simulink model "sim_nomal_regulator"  (R2019a)
settings: Solver=FixedStepAuto  StartTime=0.0  StopTime=20  FixedStep=sT  RelTol=1e-3
InitFcn:
  | sim_param;
values from neighbouring files (symbols this model uses):
  bn = 50    [robot_param.m]    (also in sim_robot_param.m)
  bt = 50    [robot_param.m]    (also in sim_robot_param.m)
  foot_x = 0.07    [robot_param.m]    (also in sim_robot_param.m)
  foot_y = 0.045    [robot_param.m]    (also in sim_robot_param.m)
  foot_z = 0.01    [robot_param.m]    (also in sim_robot_param.m)
  height_plane = 0.025    [robot_param.m]    (also in sim_robot_param.m)
  inix = [0.00 0.00]'    [param.m]    (also in sim_param.m)
  iniXzmax = 0.05    [param.m]    (also in sim_param.m)
  iniXzmin = -0.05    [param.m]    (also in sim_param.m)
  iniy = [0.00 0.00]'    [param.m]    (also in sim_param.m)
  iniYzmax = 0.0625    [param.m]    (also in sim_param.m)
  iniYzmin = -0.0625    [param.m]    (also in sim_param.m)
  kn = 5000    [robot_param.m]    (also in sim_robot_param.m)
  kt = 5000    [robot_param.m]    (also in sim_robot_param.m)
  mu_d = 0.8    [robot_param.m]    (also in sim_robot_param.m)
  mu_s = 2    [robot_param.m]    (also in sim_robot_param.m)
  plane_x = 3    [robot_param.m]    (also in sim_robot_param.m = 6)
  plane_y = 1    [robot_param.m]    (also in sim_robot_param.m)
  R = 20    [param.m]    (also in sim_param.m = 1)
  sT = 0.02    [param.m]    (also in sim_param.m = 0.001)
  torso_offset_x = 0.0    (= 0)    [robot_param.m]    (also in sim_robot_param.m)
  torso_offset_z = -torso_z/2    (= -0.05)    [robot_param.m]    (also in sim_robot_param.m)
  torso_x = 0.1    [robot_param.m]    (also in sim_robot_param.m)
  torso_y = 0.08    [robot_param.m]    (also in sim_robot_param.m)
  torso_z = 0.10    (= 0.1)    [robot_param.m]    (also in sim_robot_param.m)
  w = sqrt(g/zc)    [param.m]    (also in sim_param.m)
  zvt = 1e-3    (= 0.001)    [robot_param.m]    (also in sim_robot_param.m)
undefined symbols (not defined in the file or in its folder): Ad, Bd, Cd, Dd, DiscIntNeverNeededParam, Discrete, sigbuilder_block, Time, X, Y, Z
libraries: nesl_utility x142, sm_lib x86, cstblocks x11, ctrlSharedLib x8
(part 5 of 6)

== system sim_nomal_regulator/simulation/Robot/Right Leg/Subsystem7 ==
  Chart : Stateflow chart  TreatAsAtomicUnit=on
  Constant1 : Constant  Value=kt
  Constant2 : Constant  Value=mu_d
  Constant3 : Constant  Value=mu_s
  Constant4 : Constant  Value=zvt
  Constant5 : Constant  Value=bt
  Constant6 : Constant  Value=bn
  Constant7 : Constant  Value=kn
  External Force and Torque : sm_lib/Forces and Torques/External Force and Torque  ForceResolutionFrame=AttachedFrame  EnableForceX=off  EnableForceY=off  EnableForceZ=off  EnableForce=on  TorqueResolutionFrame=AttachedFrame  EnableTorqueX=off  EnableTorqueY=off  EnableTorqueZ=off  EnableTorque=off
  Mux : Mux  Inputs=3
  PS-Simulink Converter1 : nesl_utility/PS-Simulink Converter  PhysicalDomain=network_engine_domain  SubClassName=ps_output  LeftPortType=input  RightPortType=output  PseudoPeriodic=off  Frequencies=[]  Unit=1  AffineConversion=off
  PS-Simulink Converter2 : nesl_utility/PS-Simulink Converter  PhysicalDomain=network_engine_domain  SubClassName=ps_output  LeftPortType=input  RightPortType=output  PseudoPeriodic=off  Frequencies=[]  Unit=1  AffineConversion=off
  PS-Simulink Converter4 : nesl_utility/PS-Simulink Converter  PhysicalDomain=network_engine_domain  SubClassName=ps_output  LeftPortType=input  RightPortType=output  PseudoPeriodic=off  Frequencies=[]  Unit=m/s  AffineConversion=off
  PS-Simulink Converter5 : nesl_utility/PS-Simulink Converter  PhysicalDomain=network_engine_domain  SubClassName=ps_output  LeftPortType=input  RightPortType=output  PseudoPeriodic=off  Frequencies=[]  Unit=m/s  AffineConversion=off
  PS-Simulink dpn : nesl_utility/PS-Simulink Converter  PhysicalDomain=network_engine_domain  SubClassName=ps_output  LeftPortType=input  RightPortType=output  PseudoPeriodic=off  Frequencies=[]  Unit=m/s  AffineConversion=off
  PS-Simulink pn : nesl_utility/PS-Simulink Converter  PhysicalDomain=network_engine_domain  SubClassName=ps_output  LeftPortType=input  RightPortType=output  PseudoPeriodic=off  Frequencies=[]  Unit=1  AffineConversion=off
  Simulink-PS Converter : nesl_utility/Simulink-PS Converter  PhysicalDomain=network_engine_domain  SubClassName=ps_input  LeftPortType=input  RightPortType=output  PseudoPeriodic=off  Frequencies=[]  NoiseDistribution=none  NoiseParameters=[]  Unit=N  AffineConversion=off  FilteringAndDerivatives=provide  SimscapeFilterOrder=1  InputFilterTimeConstant=0.001  UdotUserProvided=0
  Transform Sensor : sm_lib/Frames and Transforms/Transform Sensor  MeasurementFrame=World  SenseAngle=off  SenseAxis=off  SenseAngle1=off  SenseAngle2=off  SenseAngle3=off  SenseQ=off  SenseR=off  SenseOmegaX=off  SenseOmegaY=off  SenseOmegaZ=off  SenseOmega1=off  SenseOmega2=off  SenseOmega3=off  SenseQDot=off  SenseRDot=off  SenseAlphaX=off  SenseAlphaY=off  SenseAlphaZ=off  SenseAlpha1=off  SenseAlpha2=off  SenseAlpha3=off  SenseQDDot=off  SenseRDDot=off  SenseX=on  SenseY=on  SenseZ=on  SenseRad=off  SenseAzim=off  SenseDist=off  SenseInc=off  SenseXDot=on  SenseYDot=on  SenseZDot=on  SenseRadDot=off  SenseAzimDot=off  SenseDistDot=off  SenseIncDot=off  SenseXDDot=off  SenseYDDot=off  SenseZDDot=off  SenseRadDDot=off  SenseAzimDDot=off  SenseDistDDot=off  SenseIncDDot=off
  CS : PMIOPort  Side=Right
  B : PMIOPort  Port=2  Side=Left
  mode : Outport
  Fn : Outport  Port=2
  wires:
  PS-Simulink pn/1 -> Chart/10(pn)
  Constant5/1 -> Chart/4(bt)
  Constant3/1 -> Chart/6(mu_s)
  Constant6/1 -> Chart/3(bn)
  Constant4/1 -> Chart/7(zvt)
  Constant7/1 -> Chart/1(kn)
  PS-Simulink dpn/1 -> Chart/13(dpn)
  PS-Simulink Converter1/1 -> Chart/8(px)
  PS-Simulink Converter2/1 -> Chart/9(py)
  Constant1/1 -> Chart/2(kt)
  Constant2/1 -> Chart/5(mu_d)
  Chart/3(Fn) -> Mux/3, Fn/1
  Chart/2(Fy) -> Mux/2
  PS-Simulink Converter5/1 -> Chart/12(dpy)
  Chart/1(Fx) -> Mux/1
  PS-Simulink Converter4/1 -> Chart/11(dpx)
  Chart/4(mode) -> mode/1
  Mux/1 -> Simulink-PS Converter/1
  connections:
  Transform Sensor/RConn2 -- PS-Simulink Converter1/LConn1
  Transform Sensor/RConn5 -- PS-Simulink Converter4/LConn1
  Transform Sensor/RConn6 -- PS-Simulink Converter5/LConn1
  Transform Sensor/RConn7 -- PS-Simulink dpn/LConn1
  Transform Sensor/RConn4 -- PS-Simulink pn/LConn1
  Simulink-PS Converter/RConn1 -- External Force and Torque/LConn1
  Transform Sensor/RConn3 -- PS-Simulink Converter2/LConn1
  B/RConn1 -- Transform Sensor/LConn1
  External Force and Torque/RConn1 -- Transform Sensor/RConn1 -- CS/RConn1

== system sim_nomal_regulator/simulation/Robot/Right Leg/Subsystem8 ==
  Chart : Stateflow chart  TreatAsAtomicUnit=on
  Constant1 : Constant  Value=kt
  Constant2 : Constant  Value=mu_d
  Constant3 : Constant  Value=mu_s
  Constant4 : Constant  Value=zvt
  Constant5 : Constant  Value=bt
  Constant6 : Constant  Value=bn
  Constant7 : Constant  Value=kn
  External Force and Torque : sm_lib/Forces and Torques/External Force and Torque  ForceResolutionFrame=AttachedFrame  EnableForceX=off  EnableForceY=off  EnableForceZ=off  EnableForce=on  TorqueResolutionFrame=AttachedFrame  EnableTorqueX=off  EnableTorqueY=off  EnableTorqueZ=off  EnableTorque=off
  Mux : Mux  Inputs=3
  PS-Simulink Converter1 : nesl_utility/PS-Simulink Converter  PhysicalDomain=network_engine_domain  SubClassName=ps_output  LeftPortType=input  RightPortType=output  PseudoPeriodic=off  Frequencies=[]  Unit=1  AffineConversion=off
  PS-Simulink Converter2 : nesl_utility/PS-Simulink Converter  PhysicalDomain=network_engine_domain  SubClassName=ps_output  LeftPortType=input  RightPortType=output  PseudoPeriodic=off  Frequencies=[]  Unit=1  AffineConversion=off
  PS-Simulink Converter4 : nesl_utility/PS-Simulink Converter  PhysicalDomain=network_engine_domain  SubClassName=ps_output  LeftPortType=input  RightPortType=output  PseudoPeriodic=off  Frequencies=[]  Unit=m/s  AffineConversion=off
  PS-Simulink Converter5 : nesl_utility/PS-Simulink Converter  PhysicalDomain=network_engine_domain  SubClassName=ps_output  LeftPortType=input  RightPortType=output  PseudoPeriodic=off  Frequencies=[]  Unit=m/s  AffineConversion=off
  PS-Simulink dpn : nesl_utility/PS-Simulink Converter  PhysicalDomain=network_engine_domain  SubClassName=ps_output  LeftPortType=input  RightPortType=output  PseudoPeriodic=off  Frequencies=[]  Unit=m/s  AffineConversion=off
  PS-Simulink pn : nesl_utility/PS-Simulink Converter  PhysicalDomain=network_engine_domain  SubClassName=ps_output  LeftPortType=input  RightPortType=output  PseudoPeriodic=off  Frequencies=[]  Unit=1  AffineConversion=off
  Simulink-PS Converter : nesl_utility/Simulink-PS Converter  PhysicalDomain=network_engine_domain  SubClassName=ps_input  LeftPortType=input  RightPortType=output  PseudoPeriodic=off  Frequencies=[]  NoiseDistribution=none  NoiseParameters=[]  Unit=N  AffineConversion=off  FilteringAndDerivatives=provide  SimscapeFilterOrder=1  InputFilterTimeConstant=0.001  UdotUserProvided=0
  Transform Sensor : sm_lib/Frames and Transforms/Transform Sensor  MeasurementFrame=World  SenseAngle=off  SenseAxis=off  SenseAngle1=off  SenseAngle2=off  SenseAngle3=off  SenseQ=off  SenseR=off  SenseOmegaX=off  SenseOmegaY=off  SenseOmegaZ=off  SenseOmega1=off  SenseOmega2=off  SenseOmega3=off  SenseQDot=off  SenseRDot=off  SenseAlphaX=off  SenseAlphaY=off  SenseAlphaZ=off  SenseAlpha1=off  SenseAlpha2=off  SenseAlpha3=off  SenseQDDot=off  SenseRDDot=off  SenseX=on  SenseY=on  SenseZ=on  SenseRad=off  SenseAzim=off  SenseDist=off  SenseInc=off  SenseXDot=on  SenseYDot=on  SenseZDot=on  SenseRadDot=off  SenseAzimDot=off  SenseDistDot=off  SenseIncDot=off  SenseXDDot=off  SenseYDDot=off  SenseZDDot=off  SenseRadDDot=off  SenseAzimDDot=off  SenseDistDDot=off  SenseIncDDot=off
  CS : PMIOPort  Side=Right
  B : PMIOPort  Port=2  Side=Left
  mode : Outport
  Fn : Outport  Port=2
  wires:
  PS-Simulink pn/1 -> Chart/10(pn)
  Constant5/1 -> Chart/4(bt)
  Constant3/1 -> Chart/6(mu_s)
  Constant6/1 -> Chart/3(bn)
  Constant4/1 -> Chart/7(zvt)
  Constant7/1 -> Chart/1(kn)
  PS-Simulink dpn/1 -> Chart/13(dpn)
  PS-Simulink Converter1/1 -> Chart/8(px)
  PS-Simulink Converter2/1 -> Chart/9(py)
  Constant1/1 -> Chart/2(kt)
  Constant2/1 -> Chart/5(mu_d)
  Chart/3(Fn) -> Mux/3, Fn/1
  Chart/2(Fy) -> Mux/2
  PS-Simulink Converter5/1 -> Chart/12(dpy)
  Chart/1(Fx) -> Mux/1
  PS-Simulink Converter4/1 -> Chart/11(dpx)
  Chart/4(mode) -> mode/1
  Mux/1 -> Simulink-PS Converter/1
  connections:
  Transform Sensor/RConn2 -- PS-Simulink Converter1/LConn1
  Transform Sensor/RConn5 -- PS-Simulink Converter4/LConn1
  Transform Sensor/RConn6 -- PS-Simulink Converter5/LConn1
  Transform Sensor/RConn7 -- PS-Simulink dpn/LConn1
  Transform Sensor/RConn4 -- PS-Simulink pn/LConn1
  Simulink-PS Converter/RConn1 -- External Force and Torque/LConn1
  Transform Sensor/RConn3 -- PS-Simulink Converter2/LConn1
  B/RConn1 -- Transform Sensor/LConn1
  External Force and Torque/RConn1 -- Transform Sensor/RConn1 -- CS/RConn1

== system sim_nomal_regulator/simulation/Robot/Right Leg/Subsystem9 ==
  Chart : Stateflow chart  TreatAsAtomicUnit=on
  Constant1 : Constant  Value=kt
  Constant2 : Constant  Value=mu_d
  Constant3 : Constant  Value=mu_s
  Constant4 : Constant  Value=zvt
  Constant5 : Constant  Value=bt
  Constant6 : Constant  Value=bn
  Constant7 : Constant  Value=kn
  External Force and Torque : sm_lib/Forces and Torques/External Force and Torque  ForceResolutionFrame=AttachedFrame  EnableForceX=off  EnableForceY=off  EnableForceZ=off  EnableForce=on  TorqueResolutionFrame=AttachedFrame  EnableTorqueX=off  EnableTorqueY=off  EnableTorqueZ=off  EnableTorque=off
  Mux : Mux  Inputs=3
  PS-Simulink Converter1 : nesl_utility/PS-Simulink Converter  PhysicalDomain=network_engine_domain  SubClassName=ps_output  LeftPortType=input  RightPortType=output  PseudoPeriodic=off  Frequencies=[]  Unit=1  AffineConversion=off
  PS-Simulink Converter2 : nesl_utility/PS-Simulink Converter  PhysicalDomain=network_engine_domain  SubClassName=ps_output  LeftPortType=input  RightPortType=output  PseudoPeriodic=off  Frequencies=[]  Unit=1  AffineConversion=off
  PS-Simulink Converter4 : nesl_utility/PS-Simulink Converter  PhysicalDomain=network_engine_domain  SubClassName=ps_output  LeftPortType=input  RightPortType=output  PseudoPeriodic=off  Frequencies=[]  Unit=m/s  AffineConversion=off
  PS-Simulink Converter5 : nesl_utility/PS-Simulink Converter  PhysicalDomain=network_engine_domain  SubClassName=ps_output  LeftPortType=input  RightPortType=output  PseudoPeriodic=off  Frequencies=[]  Unit=m/s  AffineConversion=off
  PS-Simulink dpn : nesl_utility/PS-Simulink Converter  PhysicalDomain=network_engine_domain  SubClassName=ps_output  LeftPortType=input  RightPortType=output  PseudoPeriodic=off  Frequencies=[]  Unit=m/s  AffineConversion=off
  PS-Simulink pn : nesl_utility/PS-Simulink Converter  PhysicalDomain=network_engine_domain  SubClassName=ps_output  LeftPortType=input  RightPortType=output  PseudoPeriodic=off  Frequencies=[]  Unit=1  AffineConversion=off
  Simulink-PS Converter : nesl_utility/Simulink-PS Converter  PhysicalDomain=network_engine_domain  SubClassName=ps_input  LeftPortType=input  RightPortType=output  PseudoPeriodic=off  Frequencies=[]  NoiseDistribution=none  NoiseParameters=[]  Unit=N  AffineConversion=off  FilteringAndDerivatives=provide  SimscapeFilterOrder=1  InputFilterTimeConstant=0.001  UdotUserProvided=0
  Transform Sensor : sm_lib/Frames and Transforms/Transform Sensor  MeasurementFrame=World  SenseAngle=off  SenseAxis=off  SenseAngle1=off  SenseAngle2=off  SenseAngle3=off  SenseQ=off  SenseR=off  SenseOmegaX=off  SenseOmegaY=off  SenseOmegaZ=off  SenseOmega1=off  SenseOmega2=off  SenseOmega3=off  SenseQDot=off  SenseRDot=off  SenseAlphaX=off  SenseAlphaY=off  SenseAlphaZ=off  SenseAlpha1=off  SenseAlpha2=off  SenseAlpha3=off  SenseQDDot=off  SenseRDDot=off  SenseX=on  SenseY=on  SenseZ=on  SenseRad=off  SenseAzim=off  SenseDist=off  SenseInc=off  SenseXDot=on  SenseYDot=on  SenseZDot=on  SenseRadDot=off  SenseAzimDot=off  SenseDistDot=off  SenseIncDot=off  SenseXDDot=off  SenseYDDot=off  SenseZDDot=off  SenseRadDDot=off  SenseAzimDDot=off  SenseDistDDot=off  SenseIncDDot=off
  CS : PMIOPort  Side=Right
  B : PMIOPort  Port=2  Side=Left
  mode : Outport
  Fn : Outport  Port=2
  wires:
  PS-Simulink pn/1 -> Chart/10(pn)
  Constant5/1 -> Chart/4(bt)
  Constant3/1 -> Chart/6(mu_s)
  Constant6/1 -> Chart/3(bn)
  Constant4/1 -> Chart/7(zvt)
  Constant7/1 -> Chart/1(kn)
  PS-Simulink dpn/1 -> Chart/13(dpn)
  PS-Simulink Converter1/1 -> Chart/8(px)
  PS-Simulink Converter2/1 -> Chart/9(py)
  Constant1/1 -> Chart/2(kt)
  Constant2/1 -> Chart/5(mu_d)
  Chart/3(Fn) -> Mux/3, Fn/1
  Chart/2(Fy) -> Mux/2
  PS-Simulink Converter5/1 -> Chart/12(dpy)
  Chart/1(Fx) -> Mux/1
  PS-Simulink Converter4/1 -> Chart/11(dpx)
  Chart/4(mode) -> mode/1
  Mux/1 -> Simulink-PS Converter/1
  connections:
  Transform Sensor/RConn2 -- PS-Simulink Converter1/LConn1
  Transform Sensor/RConn5 -- PS-Simulink Converter4/LConn1
  Transform Sensor/RConn6 -- PS-Simulink Converter5/LConn1
  Transform Sensor/RConn7 -- PS-Simulink dpn/LConn1
  Transform Sensor/RConn4 -- PS-Simulink pn/LConn1
  Simulink-PS Converter/RConn1 -- External Force and Torque/LConn1
  Transform Sensor/RConn3 -- PS-Simulink Converter2/LConn1
  B/RConn1 -- Transform Sensor/LConn1
  External Force and Torque/RConn1 -- Transform Sensor/RConn1 -- CS/RConn1

== stateflow chart sim_nomal_regulator/simulation/Robot/Left Leg/Subsystem1/Chart ==
  state No_Contact/
    (default) -> (junction 3) : {
        | mode = 1;
        |
        | Fn = 0;
        | Fx = 0; Fy = 0;
        | }
  state Sticking
    Sticking -> (junction 35) [order 1] : {
        | Fn = -(kn*pn+bn*dpn);
        | }
    (default) -> (junction 33) : {
        | mode = 4;
        |
        | Fn = -(kn*pn+bn*dpn);
        | }
    (junction 33) -> (junction 35)
    (junction 35) -> (junction 36) [order 1] : [Fn < 0]
    (junction 35) -> (junction 37) [order 2] : {
        | Fx = -(kt*(px-ax)+bt*dpx);
        | Fy = -(kt*(py-ay)+bt*dpy);
        |
        | norm_Ft = sqrt(Fx^2+Fy^2);
        | }
    (junction 36) -> (junction 41) : {
        | mode = 6;
        |
        | Fn = 0;
        | Fx = 0; Fy = 0;
        | }
    (junction 37) -> (junction 40) [order 1] : [norm_Ft > mu_s*Fn]
    (junction 37) -> (junction 38) [order 2]
    (junction 40) -> (junction 42) : {
        | mode = 5;
        |
        | Fx = mu_s*Fn*Fx/norm_Ft;
        | Fy = mu_s*Fn*Fy/norm_Ft;
        | }
    (junction 42) -> (junction 38)
    (junction 41) -> (junction 42)
    (junction 38) -> (junction 39)
  state Sliding
    Sliding -> (junction 10) [order 1] : {
        | mode = 2;
        |
        | Fn = -(kn*pn+bn*dpn);
        | }
    (default) -> (junction 8) : {
        | mode = 2;
        |
        | Fn = -(kn*pn+bn*dpn);
        | }
    (junction 8) -> (junction 10)
    (junction 10) -> (junction 11) [order 1] : [Fn < 0]
    (junction 10) -> (junction 12) [order 2] : {
        | norm_dpt = sqrt(dpx^2+dpy^2);
        | }
    (junction 11) -> (junction 17) : {
        | mode = 6;
        |
        | Fn = 0;
        | Fx = 0; Fy = 0;
        | }
    (junction 12) -> (junction 15) [order 1] : [norm_dpt <= zvt]
    (junction 12) -> (junction 13) [order 2] : {
        | Fx = -mu_d*Fn*dpx/norm_dpt;
        | Fy = -mu_d*Fn*dpy/norm_dpt;
        | }
    (junction 15) -> (junction 16) : {
        | mode = 3;
        | Fx = -mu_d*Fn*dpx/zvt;
        | Fy = -mu_d*Fn*dpy/zvt;
        |
        | ax = px;
        | ay = py;
        | }
    (junction 16) -> (junction 13)
    (junction 17) -> (junction 16)
    (junction 13) -> (junction 14)
  (default) -> No_Contact
  No_Contact -> Sliding : [pn < 0]
  Sliding -> No_Contact [order 1] : [pn >= 0]
  Sticking -> No_Contact [order 1] : [pn >= 0]
  Sliding -> Sticking [order 2] : [pn < 0 ...
      | && mode == 3]
  Sticking -> Sliding [order 2] : [pn < 0 ...
      | && (mode == 5 || mode == 6)]
  data: kn input; kt input; Fx output double; Fy output double; ax local double; ay local double; bn input; bt input; mu_d input; mu_s input; zvt input; px input; py input; pn input; dpx input; dpy input; dpn input; norm_Ft local double; norm_dpt local double; Fn output double; mode output double

== stateflow chart sim_nomal_regulator/simulation/Robot/Left Leg/Subsystem10/Chart ==
  state No_Contact/
    (default) -> (junction 3) : {
        | mode = 1;
        |
        | Fn = 0;
        | Fx = 0; Fy = 0;
        | }
  state Sticking
    Sticking -> (junction 35) [order 1] : {
        | Fn = -(kn*pn+bn*dpn);
        | }
    (default) -> (junction 33) : {
        | mode = 4;
        |
        | Fn = -(kn*pn+bn*dpn);
        | }
    (junction 33) -> (junction 35)
    (junction 35) -> (junction 36) [order 1] : [Fn < 0]
    (junction 35) -> (junction 37) [order 2] : {
        | Fx = -(kt*(px-ax)+bt*dpx);
        | Fy = -(kt*(py-ay)+bt*dpy);
        |
        | norm_Ft = sqrt(Fx^2+Fy^2);
        | }
    (junction 36) -> (junction 41) : {
        | mode = 6;
        |
        | Fn = 0;
        | Fx = 0; Fy = 0;
        | }
    (junction 37) -> (junction 40) [order 1] : [norm_Ft > mu_s*Fn]
    (junction 37) -> (junction 38) [order 2]
    (junction 40) -> (junction 42) : {
        | mode = 5;
        |
        | Fx = mu_s*Fn*Fx/norm_Ft;
        | Fy = mu_s*Fn*Fy/norm_Ft;
        | }
    (junction 42) -> (junction 38)
    (junction 41) -> (junction 42)
    (junction 38) -> (junction 39)
  state Sliding
    Sliding -> (junction 10) [order 1] : {
        | mode = 2;
        |
        | Fn = -(kn*pn+bn*dpn);
        | }
    (default) -> (junction 8) : {
        | mode = 2;
        |
        | Fn = -(kn*pn+bn*dpn);
        | }
    (junction 8) -> (junction 10)
    (junction 10) -> (junction 11) [order 1] : [Fn < 0]
    (junction 10) -> (junction 12) [order 2] : {
        | norm_dpt = sqrt(dpx^2+dpy^2);
        | }
    (junction 11) -> (junction 17) : {
        | mode = 6;
        |
        | Fn = 0;
        | Fx = 0; Fy = 0;
        | }
    (junction 12) -> (junction 15) [order 1] : [norm_dpt <= zvt]
    (junction 12) -> (junction 13) [order 2] : {
        | Fx = -mu_d*Fn*dpx/norm_dpt;
        | Fy = -mu_d*Fn*dpy/norm_dpt;
        | }
    (junction 15) -> (junction 16) : {
        | mode = 3;
        | Fx = -mu_d*Fn*dpx/zvt;
        | Fy = -mu_d*Fn*dpy/zvt;
        |
        | ax = px;
        | ay = py;
        | }
    (junction 16) -> (junction 13)
    (junction 17) -> (junction 16)
    (junction 13) -> (junction 14)
  (default) -> No_Contact
  No_Contact -> Sliding : [pn < 0]
  Sliding -> No_Contact [order 1] : [pn >= 0]
  Sticking -> No_Contact [order 1] : [pn >= 0]
  Sliding -> Sticking [order 2] : [pn < 0 ...
      | && mode == 3]
  Sticking -> Sliding [order 2] : [pn < 0 ...
      | && (mode == 5 || mode == 6)]
  data: kn input; kt input; Fx output double; Fy output double; ax local double; ay local double; bn input; bt input; mu_d input; mu_s input; zvt input; px input; py input; pn input; dpx input; dpy input; dpn input; norm_Ft local double; norm_dpt local double; Fn output double; mode output double

== stateflow chart sim_nomal_regulator/simulation/Robot/Left Leg/Subsystem11/Chart ==
  state No_Contact/
    (default) -> (junction 3) : {
        | mode = 1;
        |
        | Fn = 0;
        | Fx = 0; Fy = 0;
        | }
  state Sticking
    Sticking -> (junction 35) [order 1] : {
        | Fn = -(kn*pn+bn*dpn);
        | }
    (default) -> (junction 33) : {
        | mode = 4;
        |
        | Fn = -(kn*pn+bn*dpn);
        | }
    (junction 33) -> (junction 35)
    (junction 35) -> (junction 36) [order 1] : [Fn < 0]
    (junction 35) -> (junction 37) [order 2] : {
        | Fx = -(kt*(px-ax)+bt*dpx);
        | Fy = -(kt*(py-ay)+bt*dpy);
        |
        | norm_Ft = sqrt(Fx^2+Fy^2);
        | }
    (junction 36) -> (junction 41) : {
        | mode = 6;
        |
        | Fn = 0;
        | Fx = 0; Fy = 0;
        | }
    (junction 37) -> (junction 40) [order 1] : [norm_Ft > mu_s*Fn]
    (junction 37) -> (junction 38) [order 2]
    (junction 40) -> (junction 42) : {
        | mode = 5;
        |
        | Fx = mu_s*Fn*Fx/norm_Ft;
        | Fy = mu_s*Fn*Fy/norm_Ft;
        | }
    (junction 42) -> (junction 38)
    (junction 41) -> (junction 42)
    (junction 38) -> (junction 39)
  state Sliding
    Sliding -> (junction 10) [order 1] : {
        | mode = 2;
        |
        | Fn = -(kn*pn+bn*dpn);
        | }
    (default) -> (junction 8) : {
        | mode = 2;
        |
        | Fn = -(kn*pn+bn*dpn);
        | }
    (junction 8) -> (junction 10)
    (junction 10) -> (junction 11) [order 1] : [Fn < 0]
    (junction 10) -> (junction 12) [order 2] : {
        | norm_dpt = sqrt(dpx^2+dpy^2);
        | }
    (junction 11) -> (junction 17) : {
        | mode = 6;
        |
        | Fn = 0;
        | Fx = 0; Fy = 0;
        | }
    (junction 12) -> (junction 15) [order 1] : [norm_dpt <= zvt]
    (junction 12) -> (junction 13) [order 2] : {
        | Fx = -mu_d*Fn*dpx/norm_dpt;
        | Fy = -mu_d*Fn*dpy/norm_dpt;
        | }
    (junction 15) -> (junction 16) : {
        | mode = 3;
        | Fx = -mu_d*Fn*dpx/zvt;
        | Fy = -mu_d*Fn*dpy/zvt;
        |
        | ax = px;
        | ay = py;
        | }
    (junction 16) -> (junction 13)
    (junction 17) -> (junction 16)
    (junction 13) -> (junction 14)
  (default) -> No_Contact
  No_Contact -> Sliding : [pn < 0]
  Sliding -> No_Contact [order 1] : [pn >= 0]
  Sticking -> No_Contact [order 1] : [pn >= 0]
  Sliding -> Sticking [order 2] : [pn < 0 ...
      | && mode == 3]
  Sticking -> Sliding [order 2] : [pn < 0 ...
      | && (mode == 5 || mode == 6)]
  data: kn input; kt input; Fx output double; Fy output double; ax local double; ay local double; bn input; bt input; mu_d input; mu_s input; zvt input; px input; py input; pn input; dpx input; dpy input; dpn input; norm_Ft local double; norm_dpt local double; Fn output double; mode output double

== stateflow chart sim_nomal_regulator/simulation/Robot/Left Leg/Subsystem2/Chart ==
  state No_Contact/
    (default) -> (junction 3) : {
        | mode = 1;
        |
        | Fn = 0;
        | Fx = 0; Fy = 0;
        | }
  state Sticking
    Sticking -> (junction 35) [order 1] : {
        | Fn = -(kn*pn+bn*dpn);
        | }
    (default) -> (junction 33) : {
        | mode = 4;
        |
        | Fn = -(kn*pn+bn*dpn);
        | }
    (junction 33) -> (junction 35)
    (junction 35) -> (junction 36) [order 1] : [Fn < 0]
    (junction 35) -> (junction 37) [order 2] : {
        | Fx = -(kt*(px-ax)+bt*dpx);
        | Fy = -(kt*(py-ay)+bt*dpy);
        |
        | norm_Ft = sqrt(Fx^2+Fy^2);
        | }
    (junction 36) -> (junction 41) : {
        | mode = 6;
        |
        | Fn = 0;
        | Fx = 0; Fy = 0;
        | }
    (junction 37) -> (junction 40) [order 1] : [norm_Ft > mu_s*Fn]
    (junction 37) -> (junction 38) [order 2]
    (junction 40) -> (junction 42) : {
        | mode = 5;
        |
        | Fx = mu_s*Fn*Fx/norm_Ft;
        | Fy = mu_s*Fn*Fy/norm_Ft;
        | }
    (junction 42) -> (junction 38)
    (junction 41) -> (junction 42)
    (junction 38) -> (junction 39)
  state Sliding
    Sliding -> (junction 10) [order 1] : {
        | mode = 2;
        |
        | Fn = -(kn*pn+bn*dpn);
        | }
    (default) -> (junction 8) : {
        | mode = 2;
        |
        | Fn = -(kn*pn+bn*dpn);
        | }
    (junction 8) -> (junction 10)
    (junction 10) -> (junction 11) [order 1] : [Fn < 0]
    (junction 10) -> (junction 12) [order 2] : {
        | norm_dpt = sqrt(dpx^2+dpy^2);
        | }
    (junction 11) -> (junction 17) : {
        | mode = 6;
        |
        | Fn = 0;
        | Fx = 0; Fy = 0;
        | }
    (junction 12) -> (junction 15) [order 1] : [norm_dpt <= zvt]
    (junction 12) -> (junction 13) [order 2] : {
        | Fx = -mu_d*Fn*dpx/norm_dpt;
        | Fy = -mu_d*Fn*dpy/norm_dpt;
        | }
    (junction 15) -> (junction 16) : {
        | mode = 3;
        | Fx = -mu_d*Fn*dpx/zvt;
        | Fy = -mu_d*Fn*dpy/zvt;
        |
        | ax = px;
        | ay = py;
        | }
    (junction 16) -> (junction 13)
    (junction 17) -> (junction 16)
    (junction 13) -> (junction 14)
  (default) -> No_Contact
  No_Contact -> Sliding : [pn < 0]
  Sliding -> No_Contact [order 1] : [pn >= 0]
  Sticking -> No_Contact [order 1] : [pn >= 0]
  Sliding -> Sticking [order 2] : [pn < 0 ...
      | && mode == 3]
  Sticking -> Sliding [order 2] : [pn < 0 ...
      | && (mode == 5 || mode == 6)]
  data: kn input; kt input; Fx output double; Fy output double; ax local double; ay local double; bn input; bt input; mu_d input; mu_s input; zvt input; px input; py input; pn input; dpx input; dpy input; dpn input; norm_Ft local double; norm_dpt local double; Fn output double; mode output double

== stateflow chart sim_nomal_regulator/simulation/Robot/Left Leg/Subsystem3/Chart ==
  state No_Contact/
    (default) -> (junction 3) : {
        | mode = 1;
        |
        | Fn = 0;
        | Fx = 0; Fy = 0;
        | }
  state Sticking
    Sticking -> (junction 35) [order 1] : {
        | Fn = -(kn*pn+bn*dpn);
        | }
    (default) -> (junction 33) : {
        | mode = 4;
        |
        | Fn = -(kn*pn+bn*dpn);
        | }
    (junction 33) -> (junction 35)
    (junction 35) -> (junction 36) [order 1] : [Fn < 0]
    (junction 35) -> (junction 37) [order 2] : {
        | Fx = -(kt*(px-ax)+bt*dpx);
        | Fy = -(kt*(py-ay)+bt*dpy);
        |
        | norm_Ft = sqrt(Fx^2+Fy^2);
        | }
    (junction 36) -> (junction 41) : {
        | mode = 6;
        |
        | Fn = 0;
        | Fx = 0; Fy = 0;
        | }
    (junction 37) -> (junction 40) [order 1] : [norm_Ft > mu_s*Fn]
    (junction 37) -> (junction 38) [order 2]
    (junction 40) -> (junction 42) : {
        | mode = 5;
        |
        | Fx = mu_s*Fn*Fx/norm_Ft;
        | Fy = mu_s*Fn*Fy/norm_Ft;
        | }
    (junction 42) -> (junction 38)
    (junction 41) -> (junction 42)
    (junction 38) -> (junction 39)
  state Sliding
    Sliding -> (junction 10) [order 1] : {
        | mode = 2;
        |
        | Fn = -(kn*pn+bn*dpn);
        | }
    (default) -> (junction 8) : {
        | mode = 2;
        |
        | Fn = -(kn*pn+bn*dpn);
        | }
    (junction 8) -> (junction 10)
    (junction 10) -> (junction 11) [order 1] : [Fn < 0]
    (junction 10) -> (junction 12) [order 2] : {
        | norm_dpt = sqrt(dpx^2+dpy^2);
        | }
    (junction 11) -> (junction 17) : {
        | mode = 6;
        |
        | Fn = 0;
        | Fx = 0; Fy = 0;
        | }
    (junction 12) -> (junction 15) [order 1] : [norm_dpt <= zvt]
    (junction 12) -> (junction 13) [order 2] : {
        | Fx = -mu_d*Fn*dpx/norm_dpt;
        | Fy = -mu_d*Fn*dpy/norm_dpt;
        | }
    (junction 15) -> (junction 16) : {
        | mode = 3;
        | Fx = -mu_d*Fn*dpx/zvt;
        | Fy = -mu_d*Fn*dpy/zvt;
        |
        | ax = px;
        | ay = py;
        | }
    (junction 16) -> (junction 13)
    (junction 17) -> (junction 16)
    (junction 13) -> (junction 14)
  (default) -> No_Contact
  No_Contact -> Sliding : [pn < 0]
  Sliding -> No_Contact [order 1] : [pn >= 0]
  Sticking -> No_Contact [order 1] : [pn >= 0]
  Sliding -> Sticking [order 2] : [pn < 0 ...
      | && mode == 3]
  Sticking -> Sliding [order 2] : [pn < 0 ...
      | && (mode == 5 || mode == 6)]
  data: kn input; kt input; Fx output double; Fy output double; ax local double; ay local double; bn input; bt input; mu_d input; mu_s input; zvt input; px input; py input; pn input; dpx input; dpy input; dpn input; norm_Ft local double; norm_dpt local double; Fn output double; mode output double

== stateflow chart sim_nomal_regulator/simulation/Robot/Left Leg/Subsystem4/Chart ==
  state No_Contact/
    (default) -> (junction 3) : {
        | mode = 1;
        |
        | Fn = 0;
        | Fx = 0; Fy = 0;
        | }
  state Sticking
    Sticking -> (junction 35) [order 1] : {
        | Fn = -(kn*pn+bn*dpn);
        | }
    (default) -> (junction 33) : {
        | mode = 4;
        |
        | Fn = -(kn*pn+bn*dpn);
        | }
    (junction 33) -> (junction 35)
    (junction 35) -> (junction 36) [order 1] : [Fn < 0]
    (junction 35) -> (junction 37) [order 2] : {
        | Fx = -(kt*(px-ax)+bt*dpx);
        | Fy = -(kt*(py-ay)+bt*dpy);
        |
        | norm_Ft = sqrt(Fx^2+Fy^2);
        | }
    (junction 36) -> (junction 41) : {
        | mode = 6;
        |
        | Fn = 0;
        | Fx = 0; Fy = 0;
        | }
    (junction 37) -> (junction 40) [order 1] : [norm_Ft > mu_s*Fn]
    (junction 37) -> (junction 38) [order 2]
    (junction 40) -> (junction 42) : {
        | mode = 5;
        |
        | Fx = mu_s*Fn*Fx/norm_Ft;
        | Fy = mu_s*Fn*Fy/norm_Ft;
        | }
    (junction 42) -> (junction 38)
    (junction 41) -> (junction 42)
    (junction 38) -> (junction 39)
  state Sliding
    Sliding -> (junction 10) [order 1] : {
        | mode = 2;
        |
        | Fn = -(kn*pn+bn*dpn);
        | }
    (default) -> (junction 8) : {
        | mode = 2;
        |
        | Fn = -(kn*pn+bn*dpn);
        | }
    (junction 8) -> (junction 10)
    (junction 10) -> (junction 11) [order 1] : [Fn < 0]
    (junction 10) -> (junction 12) [order 2] : {
        | norm_dpt = sqrt(dpx^2+dpy^2);
        | }
    (junction 11) -> (junction 17) : {
        | mode = 6;
        |
        | Fn = 0;
        | Fx = 0; Fy = 0;
        | }
    (junction 12) -> (junction 15) [order 1] : [norm_dpt <= zvt]
    (junction 12) -> (junction 13) [order 2] : {
        | Fx = -mu_d*Fn*dpx/norm_dpt;
        | Fy = -mu_d*Fn*dpy/norm_dpt;
        | }
    (junction 15) -> (junction 16) : {
        | mode = 3;
        | Fx = -mu_d*Fn*dpx/zvt;
        | Fy = -mu_d*Fn*dpy/zvt;
        |
        | ax = px;
        | ay = py;
        | }
    (junction 16) -> (junction 13)
    (junction 17) -> (junction 16)
    (junction 13) -> (junction 14)
  (default) -> No_Contact
  No_Contact -> Sliding : [pn < 0]
  Sliding -> No_Contact [order 1] : [pn >= 0]
  Sticking -> No_Contact [order 1] : [pn >= 0]
  Sliding -> Sticking [order 2] : [pn < 0 ...
      | && mode == 3]
  Sticking -> Sliding [order 2] : [pn < 0 ...
      | && (mode == 5 || mode == 6)]
  data: kn input; kt input; Fx output double; Fy output double; ax local double; ay local double; bn input; bt input; mu_d input; mu_s input; zvt input; px input; py input; pn input; dpx input; dpy input; dpn input; norm_Ft local double; norm_dpt local double; Fn output double; mode output double

== stateflow chart sim_nomal_regulator/simulation/Robot/Left Leg/Subsystem7/Chart ==
  state No_Contact/
    (default) -> (junction 3) : {
        | mode = 1;
        |
        | Fn = 0;
        | Fx = 0; Fy = 0;
        | }
  state Sticking
    Sticking -> (junction 35) [order 1] : {
        | Fn = -(kn*pn+bn*dpn);
        | }
    (default) -> (junction 33) : {
        | mode = 4;
        |
        | Fn = -(kn*pn+bn*dpn);
        | }
    (junction 33) -> (junction 35)
    (junction 35) -> (junction 36) [order 1] : [Fn < 0]
    (junction 35) -> (junction 37) [order 2] : {
        | Fx = -(kt*(px-ax)+bt*dpx);
        | Fy = -(kt*(py-ay)+bt*dpy);
        |
        | norm_Ft = sqrt(Fx^2+Fy^2);
        | }
    (junction 36) -> (junction 41) : {
        | mode = 6;
        |
        | Fn = 0;
        | Fx = 0; Fy = 0;
        | }
    (junction 37) -> (junction 40) [order 1] : [norm_Ft > mu_s*Fn]
    (junction 37) -> (junction 38) [order 2]
    (junction 40) -> (junction 42) : {
        | mode = 5;
        |
        | Fx = mu_s*Fn*Fx/norm_Ft;
        | Fy = mu_s*Fn*Fy/norm_Ft;
        | }
    (junction 42) -> (junction 38)
    (junction 41) -> (junction 42)
    (junction 38) -> (junction 39)
  state Sliding
    Sliding -> (junction 10) [order 1] : {
        | mode = 2;
        |
        | Fn = -(kn*pn+bn*dpn);
        | }
    (default) -> (junction 8) : {
        | mode = 2;
        |
        | Fn = -(kn*pn+bn*dpn);
        | }
    (junction 8) -> (junction 10)
    (junction 10) -> (junction 11) [order 1] : [Fn < 0]
    (junction 10) -> (junction 12) [order 2] : {
        | norm_dpt = sqrt(dpx^2+dpy^2);
        | }
    (junction 11) -> (junction 17) : {
        | mode = 6;
        |
        | Fn = 0;
        | Fx = 0; Fy = 0;
        | }
    (junction 12) -> (junction 15) [order 1] : [norm_dpt <= zvt]
    (junction 12) -> (junction 13) [order 2] : {
        | Fx = -mu_d*Fn*dpx/norm_dpt;
        | Fy = -mu_d*Fn*dpy/norm_dpt;
        | }
    (junction 15) -> (junction 16) : {
        | mode = 3;
        | Fx = -mu_d*Fn*dpx/zvt;
        | Fy = -mu_d*Fn*dpy/zvt;
        |
        | ax = px;
        | ay = py;
        | }
    (junction 16) -> (junction 13)
    (junction 17) -> (junction 16)
    (junction 13) -> (junction 14)
  (default) -> No_Contact
  No_Contact -> Sliding : [pn < 0]
  Sliding -> No_Contact [order 1] : [pn >= 0]
  Sticking -> No_Contact [order 1] : [pn >= 0]
  Sliding -> Sticking [order 2] : [pn < 0 ...
      | && mode == 3]
  Sticking -> Sliding [order 2] : [pn < 0 ...
      | && (mode == 5 || mode == 6)]
  data: kn input; kt input; Fx output double; Fy output double; ax local double; ay local double; bn input; bt input; mu_d input; mu_s input; zvt input; px input; py input; pn input; dpx input; dpy input; dpn input; norm_Ft local double; norm_dpt local double; Fn output double; mode output double

== stateflow chart sim_nomal_regulator/simulation/Robot/Left Leg/Subsystem8/Chart ==
  state No_Contact/
    (default) -> (junction 3) : {
        | mode = 1;
        |
        | Fn = 0;
        | Fx = 0; Fy = 0;
        | }
  state Sticking
    Sticking -> (junction 35) [order 1] : {
        | Fn = -(kn*pn+bn*dpn);
        | }
    (default) -> (junction 33) : {
        | mode = 4;
        |
        | Fn = -(kn*pn+bn*dpn);
        | }
    (junction 33) -> (junction 35)
    (junction 35) -> (junction 36) [order 1] : [Fn < 0]
    (junction 35) -> (junction 37) [order 2] : {
        | Fx = -(kt*(px-ax)+bt*dpx);
        | Fy = -(kt*(py-ay)+bt*dpy);
        |
        | norm_Ft = sqrt(Fx^2+Fy^2);
        | }
    (junction 36) -> (junction 41) : {
        | mode = 6;
        |
        | Fn = 0;
        | Fx = 0; Fy = 0;
        | }
    (junction 37) -> (junction 40) [order 1] : [norm_Ft > mu_s*Fn]
    (junction 37) -> (junction 38) [order 2]
    (junction 40) -> (junction 42) : {
        | mode = 5;
        |
        | Fx = mu_s*Fn*Fx/norm_Ft;
        | Fy = mu_s*Fn*Fy/norm_Ft;
        | }
    (junction 42) -> (junction 38)
    (junction 41) -> (junction 42)
    (junction 38) -> (junction 39)
  state Sliding
    Sliding -> (junction 10) [order 1] : {
        | mode = 2;
        |
        | Fn = -(kn*pn+bn*dpn);
        | }
    (default) -> (junction 8) : {
        | mode = 2;
        |
        | Fn = -(kn*pn+bn*dpn);
        | }
    (junction 8) -> (junction 10)
    (junction 10) -> (junction 11) [order 1] : [Fn < 0]
    (junction 10) -> (junction 12) [order 2] : {
        | norm_dpt = sqrt(dpx^2+dpy^2);
        | }
    (junction 11) -> (junction 17) : {
        | mode = 6;
        |
        | Fn = 0;
        | Fx = 0; Fy = 0;
        | }
    (junction 12) -> (junction 15) [order 1] : [norm_dpt <= zvt]
    (junction 12) -> (junction 13) [order 2] : {
        | Fx = -mu_d*Fn*dpx/norm_dpt;
        | Fy = -mu_d*Fn*dpy/norm_dpt;
        | }
    (junction 15) -> (junction 16) : {
        | mode = 3;
        | Fx = -mu_d*Fn*dpx/zvt;
        | Fy = -mu_d*Fn*dpy/zvt;
        |
        | ax = px;
        | ay = py;
        | }
    (junction 16) -> (junction 13)
    (junction 17) -> (junction 16)
    (junction 13) -> (junction 14)
  (default) -> No_Contact
  No_Contact -> Sliding : [pn < 0]
  Sliding -> No_Contact [order 1] : [pn >= 0]
  Sticking -> No_Contact [order 1] : [pn >= 0]
  Sliding -> Sticking [order 2] : [pn < 0 ...
      | && mode == 3]
  Sticking -> Sliding [order 2] : [pn < 0 ...
      | && (mode == 5 || mode == 6)]
  data: kn input; kt input; Fx output double; Fy output double; ax local double; ay local double; bn input; bt input; mu_d input; mu_s input; zvt input; px input; py input; pn input; dpx input; dpy input; dpn input; norm_Ft local double; norm_dpt local double; Fn output double; mode output double

== stateflow chart sim_nomal_regulator/simulation/Robot/Left Leg/Subsystem9/Chart ==
  state No_Contact/
    (default) -> (junction 3) : {
        | mode = 1;
        |
        | Fn = 0;
        | Fx = 0; Fy = 0;
        | }
  state Sticking
    Sticking -> (junction 35) [order 1] : {
        | Fn = -(kn*pn+bn*dpn);
        | }
    (default) -> (junction 33) : {
        | mode = 4;
        |
        | Fn = -(kn*pn+bn*dpn);
        | }
    (junction 33) -> (junction 35)
    (junction 35) -> (junction 36) [order 1] : [Fn < 0]
    (junction 35) -> (junction 37) [order 2] : {
        | Fx = -(kt*(px-ax)+bt*dpx);
        | Fy = -(kt*(py-ay)+bt*dpy);
        |
        | norm_Ft = sqrt(Fx^2+Fy^2);
        | }
    (junction 36) -> (junction 41) : {
        | mode = 6;
        |
        | Fn = 0;
        | Fx = 0; Fy = 0;
        | }
    (junction 37) -> (junction 40) [order 1] : [norm_Ft > mu_s*Fn]
    (junction 37) -> (junction 38) [order 2]
    (junction 40) -> (junction 42) : {
        | mode = 5;
        |
        | Fx = mu_s*Fn*Fx/norm_Ft;
        | Fy = mu_s*Fn*Fy/norm_Ft;
        | }
    (junction 42) -> (junction 38)
    (junction 41) -> (junction 42)
    (junction 38) -> (junction 39)
  state Sliding
    Sliding -> (junction 10) [order 1] : {
        | mode = 2;
        |
        | Fn = -(kn*pn+bn*dpn);
        | }
    (default) -> (junction 8) : {
        | mode = 2;
        |
        | Fn = -(kn*pn+bn*dpn);
        | }
    (junction 8) -> (junction 10)
    (junction 10) -> (junction 11) [order 1] : [Fn < 0]
    (junction 10) -> (junction 12) [order 2] : {
        | norm_dpt = sqrt(dpx^2+dpy^2);
        | }
    (junction 11) -> (junction 17) : {
        | mode = 6;
        |
        | Fn = 0;
        | Fx = 0; Fy = 0;
        | }
    (junction 12) -> (junction 15) [order 1] : [norm_dpt <= zvt]
    (junction 12) -> (junction 13) [order 2] : {
        | Fx = -mu_d*Fn*dpx/norm_dpt;
        | Fy = -mu_d*Fn*dpy/norm_dpt;
        | }
    (junction 15) -> (junction 16) : {
        | mode = 3;
        | Fx = -mu_d*Fn*dpx/zvt;
        | Fy = -mu_d*Fn*dpy/zvt;
        |
        | ax = px;
        | ay = py;
        | }
    (junction 16) -> (junction 13)
    (junction 17) -> (junction 16)
    (junction 13) -> (junction 14)
  (default) -> No_Contact
  No_Contact -> Sliding : [pn < 0]
  Sliding -> No_Contact [order 1] : [pn >= 0]
  Sticking -> No_Contact [order 1] : [pn >= 0]
  Sliding -> Sticking [order 2] : [pn < 0 ...
      | && mode == 3]
  Sticking -> Sliding [order 2] : [pn < 0 ...
      | && (mode == 5 || mode == 6)]
  data: kn input; kt input; Fx output double; Fy output double; ax local double; ay local double; bn input; bt input; mu_d input; mu_s input; zvt input; px input; py input; pn input; dpx input; dpy input; dpn input; norm_Ft local double; norm_dpt local double; Fn output double; mode output double

== stateflow chart sim_nomal_regulator/simulation/Robot/Right Leg/Subsystem1/Chart ==
  state No_Contact/
    (default) -> (junction 3) : {
        | mode = 1;
        |
        | Fn = 0;
        | Fx = 0; Fy = 0;
        | }
  state Sticking
    Sticking -> (junction 35) [order 1] : {
        | Fn = -(kn*pn+bn*dpn);
        | }
    (default) -> (junction 33) : {
        | mode = 4;
        |
        | Fn = -(kn*pn+bn*dpn);
        | }
    (junction 33) -> (junction 35)
    (junction 35) -> (junction 36) [order 1] : [Fn < 0]
    (junction 35) -> (junction 37) [order 2] : {
        | Fx = -(kt*(px-ax)+bt*dpx);
        | Fy = -(kt*(py-ay)+bt*dpy);
        |
        | norm_Ft = sqrt(Fx^2+Fy^2);
        | }
    (junction 36) -> (junction 41) : {
        | mode = 6;
        |
        | Fn = 0;
        | Fx = 0; Fy = 0;
        | }
    (junction 37) -> (junction 40) [order 1] : [norm_Ft > mu_s*Fn]
    (junction 37) -> (junction 38) [order 2]
    (junction 40) -> (junction 42) : {
        | mode = 5;
        |
        | Fx = mu_s*Fn*Fx/norm_Ft;
        | Fy = mu_s*Fn*Fy/norm_Ft;
        | }
    (junction 42) -> (junction 38)
    (junction 41) -> (junction 42)
    (junction 38) -> (junction 39)
  state Sliding
    Sliding -> (junction 10) [order 1] : {
        | mode = 2;
        |
        | Fn = -(kn*pn+bn*dpn);
        | }
    (default) -> (junction 8) : {
        | mode = 2;
        |
        | Fn = -(kn*pn+bn*dpn);
        | }
    (junction 8) -> (junction 10)
    (junction 10) -> (junction 11) [order 1] : [Fn < 0]
    (junction 10) -> (junction 12) [order 2] : {
        | norm_dpt = sqrt(dpx^2+dpy^2);
        | }
    (junction 11) -> (junction 17) : {
        | mode = 6;
        |
        | Fn = 0;
        | Fx = 0; Fy = 0;
        | }
    (junction 12) -> (junction 15) [order 1] : [norm_dpt <= zvt]
    (junction 12) -> (junction 13) [order 2] : {
        | Fx = -mu_d*Fn*dpx/norm_dpt;
        | Fy = -mu_d*Fn*dpy/norm_dpt;
        | }
    (junction 15) -> (junction 16) : {
        | mode = 3;
        | Fx = -mu_d*Fn*dpx/zvt;
        | Fy = -mu_d*Fn*dpy/zvt;
        |
        | ax = px;
        | ay = py;
        | }
    (junction 16) -> (junction 13)
    (junction 17) -> (junction 16)
    (junction 13) -> (junction 14)
  (default) -> No_Contact
  No_Contact -> Sliding : [pn < 0]
  Sliding -> No_Contact [order 1] : [pn >= 0]
  Sticking -> No_Contact [order 1] : [pn >= 0]
  Sliding -> Sticking [order 2] : [pn < 0 ...
      | && mode == 3]
  Sticking -> Sliding [order 2] : [pn < 0 ...
      | && (mode == 5 || mode == 6)]
  data: kn input; kt input; Fx output double; Fy output double; ax local double; ay local double; bn input; bt input; mu_d input; mu_s input; zvt input; px input; py input; pn input; dpx input; dpy input; dpn input; norm_Ft local double; norm_dpt local double; Fn output double; mode output double

== stateflow chart sim_nomal_regulator/simulation/Robot/Right Leg/Subsystem10/Chart ==
  state No_Contact/
    (default) -> (junction 3) : {
        | mode = 1;
        |
        | Fn = 0;
        | Fx = 0; Fy = 0;
        | }
  state Sticking
    Sticking -> (junction 35) [order 1] : {
        | Fn = -(kn*pn+bn*dpn);
        | }
    (default) -> (junction 33) : {
        | mode = 4;
        |
        | Fn = -(kn*pn+bn*dpn);
        | }
    (junction 33) -> (junction 35)
    (junction 35) -> (junction 36) [order 1] : [Fn < 0]
    (junction 35) -> (junction 37) [order 2] : {
        | Fx = -(kt*(px-ax)+bt*dpx);
        | Fy = -(kt*(py-ay)+bt*dpy);
        |
        | norm_Ft = sqrt(Fx^2+Fy^2);
        | }
    (junction 36) -> (junction 41) : {
        | mode = 6;
        |
        | Fn = 0;
        | Fx = 0; Fy = 0;
        | }
    (junction 37) -> (junction 40) [order 1] : [norm_Ft > mu_s*Fn]
    (junction 37) -> (junction 38) [order 2]
    (junction 40) -> (junction 42) : {
        | mode = 5;
        |
        | Fx = mu_s*Fn*Fx/norm_Ft;
        | Fy = mu_s*Fn*Fy/norm_Ft;
        | }
    (junction 42) -> (junction 38)
    (junction 41) -> (junction 42)
    (junction 38) -> (junction 39)
  state Sliding
    Sliding -> (junction 10) [order 1] : {
        | mode = 2;
        |
        | Fn = -(kn*pn+bn*dpn);
        | }
    (default) -> (junction 8) : {
        | mode = 2;
        |
        | Fn = -(kn*pn+bn*dpn);
        | }
    (junction 8) -> (junction 10)
    (junction 10) -> (junction 11) [order 1] : [Fn < 0]
    (junction 10) -> (junction 12) [order 2] : {
        | norm_dpt = sqrt(dpx^2+dpy^2);
        | }
    (junction 11) -> (junction 17) : {
        | mode = 6;
        |
        | Fn = 0;
        | Fx = 0; Fy = 0;
        | }
    (junction 12) -> (junction 15) [order 1] : [norm_dpt <= zvt]
    (junction 12) -> (junction 13) [order 2] : {
        | Fx = -mu_d*Fn*dpx/norm_dpt;
        | Fy = -mu_d*Fn*dpy/norm_dpt;
        | }
    (junction 15) -> (junction 16) : {
        | mode = 3;
        | Fx = -mu_d*Fn*dpx/zvt;
        | Fy = -mu_d*Fn*dpy/zvt;
        |
        | ax = px;
        | ay = py;
        | }
    (junction 16) -> (junction 13)
    (junction 17) -> (junction 16)
    (junction 13) -> (junction 14)
  (default) -> No_Contact
  No_Contact -> Sliding : [pn < 0]
  Sliding -> No_Contact [order 1] : [pn >= 0]
  Sticking -> No_Contact [order 1] : [pn >= 0]
  Sliding -> Sticking [order 2] : [pn < 0 ...
      | && mode == 3]
  Sticking -> Sliding [order 2] : [pn < 0 ...
      | && (mode == 5 || mode == 6)]
  data: kn input; kt input; Fx output double; Fy output double; ax local double; ay local double; bn input; bt input; mu_d input; mu_s input; zvt input; px input; py input; pn input; dpx input; dpy input; dpn input; norm_Ft local double; norm_dpt local double; Fn output double; mode output double

== stateflow chart sim_nomal_regulator/simulation/Robot/Right Leg/Subsystem11/Chart ==
  state No_Contact/
    (default) -> (junction 3) : {
        | mode = 1;
        |
        | Fn = 0;
        | Fx = 0; Fy = 0;
        | }
  state Sticking
    Sticking -> (junction 35) [order 1] : {
        | Fn = -(kn*pn+bn*dpn);
        | }
    (default) -> (junction 33) : {
        | mode = 4;
        |
        | Fn = -(kn*pn+bn*dpn);
        | }
    (junction 33) -> (junction 35)
    (junction 35) -> (junction 36) [order 1] : [Fn < 0]
    (junction 35) -> (junction 37) [order 2] : {
        | Fx = -(kt*(px-ax)+bt*dpx);
        | Fy = -(kt*(py-ay)+bt*dpy);
        |
        | norm_Ft = sqrt(Fx^2+Fy^2);
        | }
    (junction 36) -> (junction 41) : {
        | mode = 6;
        |
        | Fn = 0;
        | Fx = 0; Fy = 0;
        | }
    (junction 37) -> (junction 40) [order 1] : [norm_Ft > mu_s*Fn]
    (junction 37) -> (junction 38) [order 2]
    (junction 40) -> (junction 42) : {
        | mode = 5;
        |
        | Fx = mu_s*Fn*Fx/norm_Ft;
        | Fy = mu_s*Fn*Fy/norm_Ft;
        | }
    (junction 42) -> (junction 38)
    (junction 41) -> (junction 42)
    (junction 38) -> (junction 39)
  state Sliding
    Sliding -> (junction 10) [order 1] : {
        | mode = 2;
        |
        | Fn = -(kn*pn+bn*dpn);
        | }
    (default) -> (junction 8) : {
        | mode = 2;
        |
        | Fn = -(kn*pn+bn*dpn);
        | }
    (junction 8) -> (junction 10)
    (junction 10) -> (junction 11) [order 1] : [Fn < 0]
    (junction 10) -> (junction 12) [order 2] : {
        | norm_dpt = sqrt(dpx^2+dpy^2);
        | }
    (junction 11) -> (junction 17) : {
        | mode = 6;
        |
        | Fn = 0;
        | Fx = 0; Fy = 0;
        | }
    (junction 12) -> (junction 15) [order 1] : [norm_dpt <= zvt]
    (junction 12) -> (junction 13) [order 2] : {
        | Fx = -mu_d*Fn*dpx/norm_dpt;
        | Fy = -mu_d*Fn*dpy/norm_dpt;
        | }
    (junction 15) -> (junction 16) : {
        | mode = 3;
        | Fx = -mu_d*Fn*dpx/zvt;
        | Fy = -mu_d*Fn*dpy/zvt;
        |
        | ax = px;
        | ay = py;
        | }
    (junction 16) -> (junction 13)
    (junction 17) -> (junction 16)
    (junction 13) -> (junction 14)
  (default) -> No_Contact
  No_Contact -> Sliding : [pn < 0]
  Sliding -> No_Contact [order 1] : [pn >= 0]
  Sticking -> No_Contact [order 1] : [pn >= 0]
  Sliding -> Sticking [order 2] : [pn < 0 ...
      | && mode == 3]
  Sticking -> Sliding [order 2] : [pn < 0 ...
      | && (mode == 5 || mode == 6)]
  data: kn input; kt input; Fx output double; Fy output double; ax local double; ay local double; bn input; bt input; mu_d input; mu_s input; zvt input; px input; py input; pn input; dpx input; dpy input; dpn input; norm_Ft local double; norm_dpt local double; Fn output double; mode output double

== stateflow chart sim_nomal_regulator/simulation/Robot/Right Leg/Subsystem2/Chart ==
  state No_Contact/
    (default) -> (junction 3) : {
        | mode = 1;
        |
        | Fn = 0;
        | Fx = 0; Fy = 0;
        | }
  state Sticking
    Sticking -> (junction 35) [order 1] : {
        | Fn = -(kn*pn+bn*dpn);
        | }
    (default) -> (junction 33) : {
        | mode = 4;
        |
        | Fn = -(kn*pn+bn*dpn);
        | }
    (junction 33) -> (junction 35)
    (junction 35) -> (junction 36) [order 1] : [Fn < 0]
    (junction 35) -> (junction 37) [order 2] : {
        | Fx = -(kt*(px-ax)+bt*dpx);
        | Fy = -(kt*(py-ay)+bt*dpy);
        |
        | norm_Ft = sqrt(Fx^2+Fy^2);
        | }
    (junction 36) -> (junction 41) : {
        | mode = 6;
        |
        | Fn = 0;
        | Fx = 0; Fy = 0;
        | }
    (junction 37) -> (junction 40) [order 1] : [norm_Ft > mu_s*Fn]
    (junction 37) -> (junction 38) [order 2]
    (junction 40) -> (junction 42) : {
        | mode = 5;
        |
        | Fx = mu_s*Fn*Fx/norm_Ft;
        | Fy = mu_s*Fn*Fy/norm_Ft;
        | }
    (junction 42) -> (junction 38)
    (junction 41) -> (junction 42)
    (junction 38) -> (junction 39)
  state Sliding
    Sliding -> (junction 10) [order 1] : {
        | mode = 2;
        |
        | Fn = -(kn*pn+bn*dpn);
        | }
    (default) -> (junction 8) : {
        | mode = 2;
        |
        | Fn = -(kn*pn+bn*dpn);
        | }
    (junction 8) -> (junction 10)
    (junction 10) -> (junction 11) [order 1] : [Fn < 0]
    (junction 10) -> (junction 12) [order 2] : {
        | norm_dpt = sqrt(dpx^2+dpy^2);
        | }
    (junction 11) -> (junction 17) : {
        | mode = 6;
        |
        | Fn = 0;
        | Fx = 0; Fy = 0;
        | }
    (junction 12) -> (junction 15) [order 1] : [norm_dpt <= zvt]
    (junction 12) -> (junction 13) [order 2] : {
        | Fx = -mu_d*Fn*dpx/norm_dpt;
        | Fy = -mu_d*Fn*dpy/norm_dpt;
        | }
    (junction 15) -> (junction 16) : {
        | mode = 3;
        | Fx = -mu_d*Fn*dpx/zvt;
        | Fy = -mu_d*Fn*dpy/zvt;
        |
        | ax = px;
        | ay = py;
        | }
    (junction 16) -> (junction 13)
    (junction 17) -> (junction 16)
    (junction 13) -> (junction 14)
  (default) -> No_Contact
  No_Contact -> Sliding : [pn < 0]
  Sliding -> No_Contact [order 1] : [pn >= 0]
  Sticking -> No_Contact [order 1] : [pn >= 0]
  Sliding -> Sticking [order 2] : [pn < 0 ...
      | && mode == 3]
  Sticking -> Sliding [order 2] : [pn < 0 ...
      | && (mode == 5 || mode == 6)]
  data: kn input; kt input; Fx output double; Fy output double; ax local double; ay local double; bn input; bt input; mu_d input; mu_s input; zvt input; px input; py input; pn input; dpx input; dpy input; dpn input; norm_Ft local double; norm_dpt local double; Fn output double; mode output double

== stateflow chart sim_nomal_regulator/simulation/Robot/Right Leg/Subsystem3/Chart ==
  state No_Contact/
    (default) -> (junction 3) : {
        | mode = 1;
        |
        | Fn = 0;
        | Fx = 0; Fy = 0;
        | }
  state Sticking
    Sticking -> (junction 35) [order 1] : {
        | Fn = -(kn*pn+bn*dpn);
        | }
    (default) -> (junction 33) : {
        | mode = 4;
        |
        | Fn = -(kn*pn+bn*dpn);
        | }
    (junction 33) -> (junction 35)
    (junction 35) -> (junction 36) [order 1] : [Fn < 0]
    (junction 35) -> (junction 37) [order 2] : {
        | Fx = -(kt*(px-ax)+bt*dpx);
        | Fy = -(kt*(py-ay)+bt*dpy);
        |
        | norm_Ft = sqrt(Fx^2+Fy^2);
        | }
    (junction 36) -> (junction 41) : {
        | mode = 6;
        |
        | Fn = 0;
        | Fx = 0; Fy = 0;
        | }
    (junction 37) -> (junction 40) [order 1] : [norm_Ft > mu_s*Fn]
    (junction 37) -> (junction 38) [order 2]
    (junction 40) -> (junction 42) : {
        | mode = 5;
        |
        | Fx = mu_s*Fn*Fx/norm_Ft;
        | Fy = mu_s*Fn*Fy/norm_Ft;
        | }
    (junction 42) -> (junction 38)
    (junction 41) -> (junction 42)
    (junction 38) -> (junction 39)
  state Sliding
    Sliding -> (junction 10) [order 1] : {
        | mode = 2;
        |
        | Fn = -(kn*pn+bn*dpn);
        | }
    (default) -> (junction 8) : {
        | mode = 2;
        |
        | Fn = -(kn*pn+bn*dpn);
        | }
    (junction 8) -> (junction 10)
    (junction 10) -> (junction 11) [order 1] : [Fn < 0]
    (junction 10) -> (junction 12) [order 2] : {
        | norm_dpt = sqrt(dpx^2+dpy^2);
        | }
    (junction 11) -> (junction 17) : {
        | mode = 6;
        |
        | Fn = 0;
        | Fx = 0; Fy = 0;
        | }
    (junction 12) -> (junction 15) [order 1] : [norm_dpt <= zvt]
    (junction 12) -> (junction 13) [order 2] : {
        | Fx = -mu_d*Fn*dpx/norm_dpt;
        | Fy = -mu_d*Fn*dpy/norm_dpt;
        | }
    (junction 15) -> (junction 16) : {
        | mode = 3;
        | Fx = -mu_d*Fn*dpx/zvt;
        | Fy = -mu_d*Fn*dpy/zvt;
        |
        | ax = px;
        | ay = py;
        | }
    (junction 16) -> (junction 13)
    (junction 17) -> (junction 16)
    (junction 13) -> (junction 14)
  (default) -> No_Contact
  No_Contact -> Sliding : [pn < 0]
  Sliding -> No_Contact [order 1] : [pn >= 0]
  Sticking -> No_Contact [order 1] : [pn >= 0]
  Sliding -> Sticking [order 2] : [pn < 0 ...
      | && mode == 3]
  Sticking -> Sliding [order 2] : [pn < 0 ...
      | && (mode == 5 || mode == 6)]
  data: kn input; kt input; Fx output double; Fy output double; ax local double; ay local double; bn input; bt input; mu_d input; mu_s input; zvt input; px input; py input; pn input; dpx input; dpy input; dpn input; norm_Ft local double; norm_dpt local double; Fn output double; mode output double
